simulink model "mpt_demo_rtw_explicitmpctracking"  (Simulink 7.9)
settings: Solver=FixedStepDiscrete  StartTime=0.0  StopTime=10.0  RelTol=1e-3
settings Model: Creator=mato  LastModifiedBy=mato
settings HardwareCC: ProdIntDivRoundTo=Zero  ProdEndianess=LittleEndian  ProdHWDeviceType=Generic->32-bit x86 compatible
settings RTWCC: SystemTargetFile=rtwin.tlc  TemplateMakefile=rtwin.tmf  Description=Real-Time Windows Target  ProcessScript=rtwin_make_rtw_hook  RTWCompilerOptimization=On
settings CodeAppCC: MaxIdLength=95
settings TargetCC: TargetLibSuffix=_rtwin.lib  TargetPreCompLibLocation=C:\Program Files\MATLAB\R2012a\toolbox\rtw\targets\rtwin\lib\win32  CodeReplacementLibrary=ANSI_C  CodeExecutionProfiling=off  IsPILTarget=off  EnableShiftOperators=on  PortableWordSizes=off
settings CustomProperty: DataType=string  Value=C:/PROGRA~1/MATLAB/R2012a/toolbox/rtw/targets/rtwin

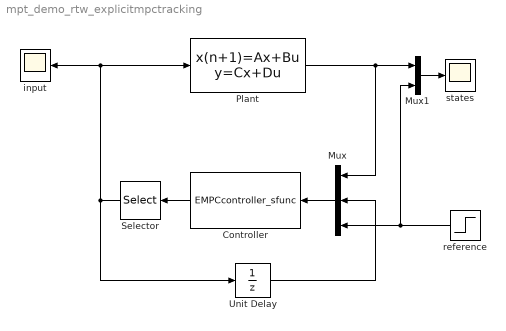
== system mpt_demo_rtw_explicitmpctracking ==
  Controller : S-Function  FunctionName=EMPCcontroller_sfunc  EnableBusSupport=off
  Mux : Mux  Inputs=3
  Mux1 : Mux  Inputs=2
  Plant : DiscreteStateSpace  A="[   0.5403   -0.8415; 0.8415    0.5403];"  B=[ -0.4597; 0.8415];  C=eye(2)  D=[0;0]  X0=[0;0]
  Selector : Selector  InputPortWidth=4  IndexOptions=Index vector (dialog)  Indices=1  OutputSizes=1
  Unit Delay : UnitDelay  SampleTime=-1
  input : Scope
  reference : Step  SampleTime=0
  states : Scope
  wires:
  Controller/1 -> Selector/1
  Mux/1 -> Controller/1
  reference/1 -> Mux1/2, Mux/3
  Mux1/1 -> states/1
  Plant/1 -> Mux/1, Mux1/1
  Selector/1 -> Plant/1, input/1, Unit Delay/1
  Unit Delay/1 -> Mux/2
